simulink model "test_2CAN"  (R2017b)
settings: Solver=FixedStepDiscrete  StartTime=0.0  StopTime=Inf  FixedStep=Ts  RelTol=1e-3
PreLoadFcn:
  | Ts = 0.01;
PostLoadFcn:
  | , if any(exist('dsrtsu_mdlpostloadfcn', 'file') == [2, 3, 6]), try dsrtsu_mdlpostloadfcn('Execute', bdroot); catch fprintf('Error in PostLoadFcn (dsrtsu_mdlpostloadfcn) for model "%s":\n %s\n', bdroot, lasterr); end, end,
libraries: rtican x19, simulink x6, rti1401lib_adc_type4 x3
(part 6 of 6)

== system test_2CAN/__Controller/Driving Wheel Control/Subsystem ==
  note: wheel N*m
  note: mN*m
  note: Motor N*m
  N*m : Inport
  Constant : Constant  Value=55.08
  Constant1 : Constant  Value=1000
  Constant2 : Constant  Value=190
  Divide : Product  Inputs=*/
  Divide1 : Product  Inputs=**
  Divide3 : Product  Inputs=*/
  Gain : Gain  Gain=1000
  Gain1 : Gain  Gain=-1
  Saturation Dynamic : simulink/Discontinuities/Saturation Dynamic  OutMin=[]  OutMax=[]  OutDataTypeStr=Inherit: Same as second input  OutDataType=fixdt(1, 16)  OutScaling=2^-10  DoSatur=off
  Target Torque : Outport
  wires:
  Constant2/1 -> Divide3/2
  Gain/1 -> Target Torque/1
  Divide/1 -> Gain/1
  N*m/1 -> Divide3/1
  Divide1/1 -> Saturation Dynamic/2
  Constant1/1 -> Divide1/2
  Divide3/1 -> Divide1/1
  Saturation Dynamic/1 -> Divide/1
  Gain1/1 -> Saturation Dynamic/3
  Constant/1 -> Saturation Dynamic/1, Gain1/1, Divide/2

== system test_2CAN/__Data Plotting/__Reference_Plot/If Action Subsystem4 ==
  In1 : Inport
  Action Port : ActionPort  ActionType=elseif
  Out1 : Outport
  wires:
  In1/1 -> Out1/1

== system test_2CAN/__Data Plotting/__Reference_Plot/If Action Subsystem5 ==
  note: rpm
  note: Motor rad/s
  note: Wheel rad/s
  In1 : Inport
  Action Port : ActionPort  ActionType=then
  Constant1 : Constant  Value=2*pi
  Constant5 : Constant  Value=60
  N_dri : Constant  Value=190
  Product : Product  Inputs=*/
  Product1 : Product  Inputs=**
  Product2 : Product  Inputs=*/
  Out1 : Outport
  wires:
  Constant1/1 -> Product/1
  Constant5/1 -> Product/2
  In1/1 -> Product1/1
  Product/1 -> Product1/2
  Product1/1 -> Product2/1
  N_dri/1 -> Product2/2
  Product2/1 -> Out1/1

== system test_2CAN/__Data Plotting/__Reference_Plot/If Action Subsystem6 ==
  In1 : Inport
  Action Port : ActionPort  ActionType=else
  Out1 : Outport
  wires:
  In1/1 -> Out1/1

== system test_2CAN/__Data Plotting/__Sensor_Plot/Subsystem ==
  Voltage : Inport
  Ample Gain : Constant  Value=600
  Constant : Constant  Value=300
  Divide1 : Product  Inputs=**
  Divide2 : Product  Inputs=**
  Divide3 : Product  Inputs=*/
  Divide4 : Product  Inputs=**
  V : Constant  Value=0.0161
  N : Outport
  wires:
  Constant/1 -> Divide2/2
  V/1 -> Divide1/1
  Ample Gain/1 -> Divide1/2
  Divide2/1 -> Divide3/1
  Divide1/1 -> Divide3/2
  Voltage/1 -> Divide2/1
  Divide3/1 -> Divide4/1
  [Load_cell_Gain] -> Divide4/2
  Divide4/1 -> N/1

== system test_2CAN/__Data Plotting/__Sensor_Plot/Subsystem1 ==
  Voltage : Inport
  Ample Gain : Constant  Value=600
  Constant : Constant  Value=300
  Constant1 : Constant  Commented=on  Value=30
  Divide1 : Product  Inputs=**
  Divide2 : Product  Inputs=**
  Divide3 : Product  Inputs=*/
  Divide4 : Product  Commented=on  Inputs=**
  Divide5 : Product  Inputs=**
  V : Constant  Value=0.0161
  N : Outport
  wires:
  Constant/1 -> Divide2/2
  V/1 -> Divide1/1
  Ample Gain/1 -> Divide1/2
  Divide2/1 -> Divide3/1
  Divide1/1 -> Divide3/2
  Constant1/1 -> Divide4/2
  Voltage/1 -> Divide2/1
  Divide3/1 -> Divide5/1
  Divide5/1 -> N/1
  [Load_cell_Gain] -> Divide5/2

== system test_2CAN/__System_Setting/Subsystem/ID_Mode ==
  Action Port : ActionPort  ActionType=else
  Constant : Constant  Value=10
  Constant1 : Constant  Value=3
  Mode : Outport
  Out2 : Outport  Port=2
  wires:
  Constant1/1 -> Out2/1
  Constant/1 -> Mode/1

== system test_2CAN/__System_Setting/Subsystem/Torque Mode ==
  Action Port : ActionPort  ActionType=elseif
  Constant : Constant  Value=10
  Constant1 : Constant
  Mode : Outport
  Out2 : Outport  Port=2
  wires:
  Constant/1 -> Mode/1
  Constant1/1 -> Out2/1

== system test_2CAN/__System_Setting/Subsystem/Torque Mode1 ==
  Action Port : ActionPort  ActionType=elseif
  Constant : Constant  Value=10
  Constant1 : Constant  Value=2
  Mode : Outport
  Out2 : Outport  Port=2
  wires:
  Constant/1 -> Mode/1
  Constant1/1 -> Out2/1

== system test_2CAN/__System_Setting/Subsystem/Velocity Mode ==
  Action Port : ActionPort  ActionType=then
  Constant : Constant  Value=9
  Out1 : Outport
  wires:
  Constant/1 -> Out1/1

== system test_2CAN/RTI Data/RTI Data Store/RTI Data Store/RTI Data Store ==
  RTI Data Store : Subsystem  mask(RTI_DATA_STORE){}
      mask help:
      | RTI Data Store Block. This block is used by RTI to store internal model dependent data. Deleting this block will result in data loss.
      |
      | NEVER DELETE, COPY, OR MODIFY THIS BLOCK!
      mask Help:
      | RTI Data Store Block. This block is used by RTI to store internal model dependent data. Deleting this block will result in data loss.
      | 
      | NEVER DELETE, COPY, OR MODIFY THIS BLOCK!
      mask Display: text(0.5, 0.5, ' ', 'HorizontalAlignment', 'center');

== system test_2CAN/_Reference/_dri_motor_ref/Driving_Torque_Ref/If Action Subsystem1 ==
  In1 : Inport
  Action Port : ActionPort  ActionType=elseif
  Out1 : Outport
  wires:
  In1/1 -> Out1/1

== system test_2CAN/_Reference/_dri_motor_ref/Driving_Torque_Ref/If Action Subsystem2 ==
  In1 : Inport
  Action Port : ActionPort  ActionType=then
  Out1 : Outport
  wires:
  In1/1 -> Out1/1

== system test_2CAN/_Reference/_dri_motor_ref/Driving_Torque_Ref/If Action Subsystem3 ==
  In1 : Inport
  Action Port : ActionPort  ActionType=else
  Out1 : Outport
  wires:
  In1/1 -> Out1/1

== system test_2CAN/_Reference/_dri_motor_ref/Driving_Torque_Ref/LPF ==
  note: LPF : tau = 1/(2*pi*fc)
  note: y(n) = [Ts*{x(n)+x(n-1)}+(2*tau-Ts)*y(n-1)]/(2*tau+Ts)
  note: H(s) = 1/(tau*s+1)
  note: s = 2/Ts*(z-1)/(z+1)
  In : Inport
  fc : Inport  Port=2
  Constant : Constant  Value=Ts  SampleTime=Ts
  Constant1 : Constant  SampleTime=Ts
  Product1 : Product  Inputs=*/  RndMeth=Zero
  Product11 : Product  RndMeth=Zero
  Product2 : Product  Inputs=*/  RndMeth=Zero
  Sum1 : Sum  Inputs=+-  SaturateOnIntegerOverflow=on  InputSameDT=on  OutDataTypeStr=Inherit: Same as first input
  Sum2 : Sum  SaturateOnIntegerOverflow=on  InputSameDT=on  OutDataTypeStr=Inherit: Same as first input
  Sum3 : Sum  SaturateOnIntegerOverflow=on  InputSameDT=on  OutDataTypeStr=Inherit: Same as first input
  Sum4 : Sum  SaturateOnIntegerOverflow=on  InputSameDT=on  OutDataTypeStr=Inherit: Same as first input
  d : UnitDelay  SampleTime=Ts
  d1 : UnitDelay  SampleTime=Ts
  gain : Gain  Gain=Ts  SaturateOnIntegerOverflow=on  OutDataTypeStr=Inherit: Same as input  ParamDataTypeStr=Inherit: Same as input
  gain1 : Gain  Gain=2  SaturateOnIntegerOverflow=on  OutDataTypeStr=Inherit: Same as input  ParamDataTypeStr=Inherit: Same as input
  gain2 : Gain  Gain=2*pi  SaturateOnIntegerOverflow=on  OutDataTypeStr=Inherit: Same as input  ParamDataTypeStr=Inherit: Same as input
  Out : Outport
  wires:
  In/1 -> Sum3/1, d1/1
  d1/1 -> Sum3/2
  Sum3/1 -> gain/1
  gain/1 -> Sum2/1
  Product11/1 -> Sum2/2
  Sum1/1 -> Product11/1
  Constant/1 -> Sum1/2, Sum4/2
  fc/1 -> gain2/1
  gain1/1 -> Sum1/1, Sum4/1
  d/1 -> Product11/2
  Sum2/1 -> Product1/1
  Sum4/1 -> Product1/2
  Product1/1 -> Out/1, d/1
  Product2/1 -> gain1/1
  Constant1/1 -> Product2/1
  gain2/1 -> Product2/2

== system test_2CAN/_Reference/_dri_motor_ref/Driving_Vel_Ref/LPF ==
  note: LPF : tau = 1/(2*pi*fc)
  note: y(n) = [Ts*{x(n)+x(n-1)}+(2*tau-Ts)*y(n-1)]/(2*tau+Ts)
  note: H(s) = 1/(tau*s+1)
  note: s = 2/Ts*(z-1)/(z+1)
  In : Inport
  fc : Inport  Port=2
  Constant : Constant  Value=Ts  SampleTime=Ts
  Constant1 : Constant  SampleTime=Ts
  Product1 : Product  Inputs=*/  RndMeth=Zero
  Product11 : Product  RndMeth=Zero
  Product2 : Product  Inputs=*/  RndMeth=Zero
  Sum1 : Sum  Inputs=+-  SaturateOnIntegerOverflow=on  InputSameDT=on  OutDataTypeStr=Inherit: Same as first input
  Sum2 : Sum  SaturateOnIntegerOverflow=on  InputSameDT=on  OutDataTypeStr=Inherit: Same as first input
  Sum3 : Sum  SaturateOnIntegerOverflow=on  InputSameDT=on  OutDataTypeStr=Inherit: Same as first input
  Sum4 : Sum  SaturateOnIntegerOverflow=on  InputSameDT=on  OutDataTypeStr=Inherit: Same as first input
  d : UnitDelay  SampleTime=Ts
  d1 : UnitDelay  SampleTime=Ts
  gain : Gain  Gain=Ts  SaturateOnIntegerOverflow=on  OutDataTypeStr=Inherit: Same as input  ParamDataTypeStr=Inherit: Same as input
  gain1 : Gain  Gain=2  SaturateOnIntegerOverflow=on  OutDataTypeStr=Inherit: Same as input  ParamDataTypeStr=Inherit: Same as input
  gain2 : Gain  Gain=2*pi  SaturateOnIntegerOverflow=on  OutDataTypeStr=Inherit: Same as input  ParamDataTypeStr=Inherit: Same as input
  Out : Outport
  wires:
  In/1 -> Sum3/1, d1/1
  d1/1 -> Sum3/2
  Sum3/1 -> gain/1
  gain/1 -> Sum2/1
  Product11/1 -> Sum2/2
  Sum1/1 -> Product11/1
  Constant/1 -> Sum1/2, Sum4/2
  fc/1 -> gain2/1
  gain1/1 -> Sum1/1, Sum4/1
  d/1 -> Product11/2
  Sum2/1 -> Product1/1
  Sum4/1 -> Product1/2
  Product1/1 -> Out/1, d/1
  Product2/1 -> gain1/1
  Constant1/1 -> Product2/1
  gain2/1 -> Product2/2

== system test_2CAN/__Controller/Driving Wheel Control/DOB(omega)/Dot2 ==
  note: Dot
  in : Inport
  Sum1 : Sum  Inputs=+-  SaturateOnIntegerOverflow=on  InputSameDT=on  OutDataTypeStr=Inherit: Same as first input
  Sum2 : Sum  Inputs=+-  SaturateOnIntegerOverflow=on  InputSameDT=on  OutDataTypeStr=Inherit: Same as first input
  d : UnitDelay  SampleTime=Ts
  d1 : UnitDelay  SampleTime=Ts
  gain : Gain  Gain=2/Ts  SaturateOnIntegerOverflow=on  OutDataTypeStr=Inherit: Same as input  ParamDataTypeStr=Inherit: Same as input
  out : Outport
  wires:
  Sum1/1 -> d1/1, out/1
  d1/1 -> Sum1/2
  Sum2/1 -> gain/1
  in/1 -> d/1, Sum2/1
  d/1 -> Sum2/2
  gain/1 -> Sum1/1

== system test_2CAN/__Controller/Driving Wheel Control/DOB(omega)/LPF ==
  note: LPF : tau = 1/(2*pi*fc)
  note: y(n) = [Ts*{x(n)+x(n-1)}+(2*tau-Ts)*y(n-1)]/(2*tau+Ts)
  note: H(s) = 1/(tau*s+1)
  note: s = 2/Ts*(z-1)/(z+1)
  In : Inport
  fc : Inport  Port=2
  Constant : Constant  Value=Ts  SampleTime=Ts
  Constant1 : Constant  SampleTime=Ts
  Product1 : Product  Inputs=*/  RndMeth=Zero
  Product11 : Product  RndMeth=Zero
  Product2 : Product  Inputs=*/  RndMeth=Zero
  Sum1 : Sum  Inputs=+-  SaturateOnIntegerOverflow=on  InputSameDT=on  OutDataTypeStr=Inherit: Same as first input
  Sum2 : Sum  SaturateOnIntegerOverflow=on  InputSameDT=on  OutDataTypeStr=Inherit: Same as first input
  Sum3 : Sum  SaturateOnIntegerOverflow=on  InputSameDT=on  OutDataTypeStr=Inherit: Same as first input
  Sum4 : Sum  SaturateOnIntegerOverflow=on  InputSameDT=on  OutDataTypeStr=Inherit: Same as first input
  d : UnitDelay  SampleTime=Ts
  d1 : UnitDelay  SampleTime=Ts
  gain : Gain  Gain=Ts  SaturateOnIntegerOverflow=on  OutDataTypeStr=Inherit: Same as input  ParamDataTypeStr=Inherit: Same as input
  gain1 : Gain  Gain=2  SaturateOnIntegerOverflow=on  OutDataTypeStr=Inherit: Same as input  ParamDataTypeStr=Inherit: Same as input
  gain2 : Gain  Gain=2*pi  SaturateOnIntegerOverflow=on  OutDataTypeStr=Inherit: Same as input  ParamDataTypeStr=Inherit: Same as input
  Out : Outport
  wires:
  In/1 -> Sum3/1, d1/1
  d1/1 -> Sum3/2
  Sum3/1 -> gain/1
  gain/1 -> Sum2/1
  Product11/1 -> Sum2/2
  Sum1/1 -> Product11/1
  Constant/1 -> Sum1/2, Sum4/2
  fc/1 -> gain2/1
  gain1/1 -> Sum1/1, Sum4/1
  d/1 -> Product11/2
  Sum2/1 -> Product1/1
  Sum4/1 -> Product1/2
  Product1/1 -> Out/1, d/1
  Product2/1 -> gain1/1
  Constant1/1 -> Product2/1
  gain2/1 -> Product2/2

== system test_2CAN/__Controller/Driving Wheel Control/Feedforward(omega)/Dot2 ==
  note: Dot
  in : Inport
  Sum1 : Sum  Inputs=+-  SaturateOnIntegerOverflow=on  InputSameDT=on  OutDataTypeStr=Inherit: Same as first input
  Sum2 : Sum  Inputs=+-  SaturateOnIntegerOverflow=on  InputSameDT=on  OutDataTypeStr=Inherit: Same as first input
  d : UnitDelay  SampleTime=Ts
  d1 : UnitDelay  SampleTime=Ts
  gain : Gain  Gain=2/Ts  SaturateOnIntegerOverflow=on  OutDataTypeStr=Inherit: Same as input  ParamDataTypeStr=Inherit: Same as input
  out : Outport
  wires:
  Sum1/1 -> d1/1, out/1
  d1/1 -> Sum1/2
  Sum2/1 -> gain/1
  in/1 -> d/1, Sum2/1
  d/1 -> Sum2/2
  gain/1 -> Sum1/1

== system test_2CAN/__Controller/Driving Wheel Control/Feedforward(omega)/LPF ==
  note: LPF : tau = 1/(2*pi*fc)
  note: y(n) = [Ts*{x(n)+x(n-1)}+(2*tau-Ts)*y(n-1)]/(2*tau+Ts)
  note: H(s) = 1/(tau*s+1)
  note: s = 2/Ts*(z-1)/(z+1)
  In : Inport
  fc : Inport  Port=2
  Constant : Constant  Value=Ts  SampleTime=Ts
  Constant1 : Constant  SampleTime=Ts
  Product1 : Product  Inputs=*/  RndMeth=Zero
  Product11 : Product  RndMeth=Zero
  Product2 : Product  Inputs=*/  RndMeth=Zero
  Sum1 : Sum  Inputs=+-  SaturateOnIntegerOverflow=on  InputSameDT=on  OutDataTypeStr=Inherit: Same as first input
  Sum2 : Sum  SaturateOnIntegerOverflow=on  InputSameDT=on  OutDataTypeStr=Inherit: Same as first input
  Sum3 : Sum  SaturateOnIntegerOverflow=on  InputSameDT=on  OutDataTypeStr=Inherit: Same as first input
  Sum4 : Sum  SaturateOnIntegerOverflow=on  InputSameDT=on  OutDataTypeStr=Inherit: Same as first input
  d : UnitDelay  SampleTime=Ts
  d1 : UnitDelay  SampleTime=Ts
  gain : Gain  Gain=Ts  SaturateOnIntegerOverflow=on  OutDataTypeStr=Inherit: Same as input  ParamDataTypeStr=Inherit: Same as input
  gain1 : Gain  Gain=2  SaturateOnIntegerOverflow=on  OutDataTypeStr=Inherit: Same as input  ParamDataTypeStr=Inherit: Same as input
  gain2 : Gain  Gain=2*pi  SaturateOnIntegerOverflow=on  OutDataTypeStr=Inherit: Same as input  ParamDataTypeStr=Inherit: Same as input
  Out : Outport
  wires:
  In/1 -> Sum3/1, d1/1
  d1/1 -> Sum3/2
  Sum3/1 -> gain/1
  gain/1 -> Sum2/1
  Product11/1 -> Sum2/2
  Sum1/1 -> Product11/1
  Constant/1 -> Sum1/2, Sum4/2
  fc/1 -> gain2/1
  gain1/1 -> Sum1/1, Sum4/1
  d/1 -> Product11/2
  Sum2/1 -> Product1/1
  Sum4/1 -> Product1/2
  Product1/1 -> Out/1, d/1
  Product2/1 -> gain1/1
  Constant1/1 -> Product2/1
  gain2/1 -> Product2/2

== system test_2CAN/__Controller/Driving Wheel Control/Poleplacement(PI)1/Integrator1 ==
  note: Integrator
  in : Inport
  "Off : 0 On : 1" : Inport  Port=2
  Divide : Product  Inputs=**
  Sum1 : Sum  SaturateOnIntegerOverflow=on  InputSameDT=on  OutDataTypeStr=Inherit: Same as first input
  Sum2 : Sum  SaturateOnIntegerOverflow=on  InputSameDT=on  OutDataTypeStr=Inherit: Same as first input
  d : UnitDelay  SampleTime=Ts
  d1 : UnitDelay  SampleTime=Ts
  gain : Gain  Gain=Ts/2  SaturateOnIntegerOverflow=on  OutDataTypeStr=Inherit: Same as input  ParamDataTypeStr=Inherit: Same as input
  out : Outport
  wires:
  gain/1 -> Sum2/1
  Sum1/1 -> gain/1
  d1/1 -> Sum1/2
  in/1 -> d1/1, Sum1/1
  Sum2/1 -> Divide/1, out/1
  d/1 -> Sum2/2
  Divide/1 -> d/1
  "Off : 0 On : 1"/1 -> Divide/2

== system test_2CAN/RTI Data/RTI Data Store/RTI Data Store/RTI Data Store/RTI Data Store ==

== matlab function test_2CAN/_Reference/_dri_motor_ref/Driving_Torque_Ref/MATLAB Function ==
  data: t input; y output; f input; mag input; flag input
function y = fcn(t, f, mag, flag)

    % 상태 보존을 위한 persistent 변수 선언
    persistent current_f next_f current_mag next_mag t0 prev_phase

    if flag == 0
        % 초기화 상태: 출력 0과 함께 persistent 변수 초기화
        y = 0;
        current_f = f;    % 현재 사용 주파수를 입력 f로 설정
        next_f = f;       % 다음 주기 적용될 주파수도 우선 입력 f로 설정
        current_mag = mag;  % 현재 사용 진폭 설정
        next_mag = mag;     % 다음 주기 적용될 진폭도 우선 입력 mag로 설정
        t0 = t;            % 현재 시간을 주기의 시작 시간으로 저장
        prev_phase = 0;    % 이전 위상 값 초기화
    else  % flag == 1인 경우(정상 운용)
        % persistent 변수 초기화가 안된 경우 초기화 수행
        if isempty(current_f)
            current_f = f;
            next_f = f;
            current_mag = mag;
            next_mag = mag;
            t0 = t;
            prev_phase = 0;
        end

        % 주파수(f)와 진폭(mag)이 현재 주파수와 다르면 next_f와 next_mag에 저장
        if f ~= current_f
            next_f = f;
        end
        if mag ~= current_mag
            next_mag = mag;
        end

        % 현재 주기에서의 위상 계산: 현재 주파수(current_f)와 현재 진폭(current_mag)로 진행
        phase = 2 * pi * current_f * (t - t0);
        y = current_mag * sin(phase);  % 진폭을 고려하여 사인파 출력

        % 현재 위상의 modulo 계산 (0 ~ 2*pi 사이)
        current_mod = mod(phase, 2*pi);

        % 위상의 wrap-around 감지: 이전 위상(prev_phase)보다 작아진 경우 주기 종료
        if current_mod < prev_phase
            % 한 주기가 완료되었으므로, 다음 주기에는 next_f와 next_mag을 사용
            current_f = next_f;
            current_mag = next_mag;
            t0 = t;  % 새로운 주기의 시작 시간 업데이트
        end

        % 이전 위상 값 갱신
        prev_phase = current_mod;
    end
end
